simulink model "Ejercicio1_DB"  (R2023a)
settings: Solver=VariableStepAuto  StartTime=0.0  StopTime=3.5  RelTol=1e-3
values from neighbouring files (symbols this model uses):
  a1 = 60    [Ejercicio1.m]
  a2 = 4    [Ejercicio1.m]
  a3 = 11    [Ejercicio1.m]
  b0 = 1.5    [Ejercicio1.m]
  g0 = 1/(MC*inv(MB*K-MA)*MB)    [Ejercicio1.m]
  K = acker(MA,MB,P_LC)    [Ejercicio1.m]
settings Model: Creator=54115  LastModifiedBy=franc
settings SolverCC: AlgebraicLoopSolver=TrustRegion
settings DebuggingCC: UnconnectedInputMsg=warning  UnconnectedOutputMsg=warning  UnconnectedLineMsg=warning
settings ModelReferenceCC: EnableRefExpFcnMdlSchedulingChecks=on

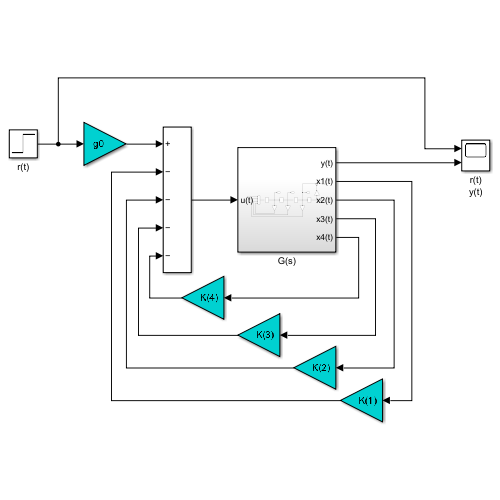
[thumbnail: Simulink's stored preview of the top-level diagram]
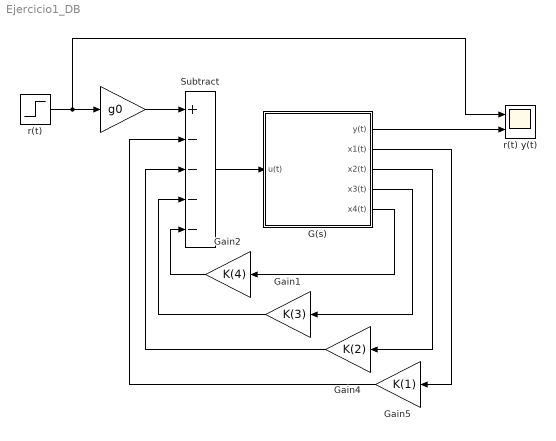
== system Ejercicio1_DB ==
  " " : Gain  Gain=g0
  G(s) : Subsystem
  Gain1 : Gain  Gain=K(3)
  Gain2 : Gain  Gain=K(4)
  Gain4 : Gain  Gain=K(2)
  Gain5 : Gain  Gain=K(1)
  Subtract : Sum  Inputs=+----
  r(t) : Step  Time=0  SampleTime=0
  r(t) y(t) : Scope  NumInputPorts=2
  wires:
  Subtract/1 -> G(s)/1(u(t))
  " "/1 -> Subtract/1
  r(t)/1 -> r(t) y(t)/1, " "/1
  G(s)/1(y(t)) -> r(t) y(t)/2
  G(s)/5(x4(t)) -> Gain2/1
  G(s)/4(x3(t)) -> Gain1/1
  G(s)/3(x2(t)) -> Gain4/1
  G(s)/2(x1(t)) -> Gain5/1
  Gain2/1 -> Subtract/5
  Gain1/1 -> Subtract/4
  Gain4/1 -> Subtract/3
  Gain5/1 -> Subtract/2

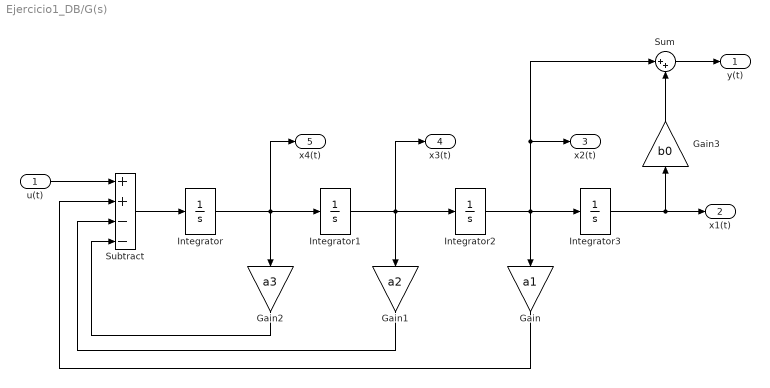
== system Ejercicio1_DB/G(s) ==
  u(t) : Inport
  Gain : Gain  Gain=a1
  Gain1 : Gain  Gain=a2
  Gain2 : Gain  Gain=a3
  Gain3 : Gain  Gain=b0
  Integrator{,1..3} (4 alike) : Integrator
  Subtract : Sum  Inputs=++--
  Sum : Sum  Inputs=|++
  y(t) : Outport
  x1(t) : Outport  Port=2
  x2(t) : Outport  Port=3
  x3(t) : Outport  Port=4
  x4(t) : Outport  Port=5
  wires:
  Integrator1/1 -> Integrator2/1, x3(t)/1, Gain1/1
  Gain3/1 -> Sum/2
  Integrator2/1 -> Integrator3/1, x2(t)/1, Sum/1, Gain/1
  Gain/1 -> Subtract/2
  Sum/1 -> y(t)/1
  Gain2/1 -> Subtract/4
  Integrator/1 -> x4(t)/1, Gain2/1, Integrator1/1
  u(t)/1 -> Subtract/1
  Gain1/1 -> Subtract/3
  Subtract/1 -> Integrator/1
  Integrator3/1 -> x1(t)/1, Gain3/1
